simulink model "SatSIM_revAgustus16_01_R2013a"  (R2013a)
settings: Solver=ode15s  StartTime=0.0  StopTime=6000  RelTol=1e-3
values from neighbouring files (symbols this model uses):
  dfy = d    [dfy.m]
  s = sin(ir)    [B_dipole_June16_2.m]    (also in LTC_to_NED.m = sin(e); LTC_to_NED_edit.m = sin(e); TimeConverter.m = fix(sec); read_epoch.m = ((e-h)*60)-min)
undefined symbols (not defined in the file or in its folder): B_dipole_June16_2, DCM_ROI, deg, Earth_MagField_may16_Rev4, InertiaMoment3, LTC_to_NED_edit, rad, read_epochS, sec_to_ymdhms2, SimpleB5
libraries: aerolibconvert2 x13, aerolibutil x7, aerolibtransform2 x4, dspmtrx3 x3, vrlib x2, aerolibanim x1
(part 1 of 2)
settings Model: Creator=Ali Muksin  LastModifiedBy=Ali Muksin
settings DebuggingCC: UnderspecifiedInitializationDetection=Simplified  MergeDetectMultiDrivingBlocksExec=error  SolverPrmCheckMsg=none  FrameProcessingCompatibilityMsg=error  StateNameClashWarn=none
settings GRTTargetCC: CodeReplacementLibrary=C89/C90 (ANSI)

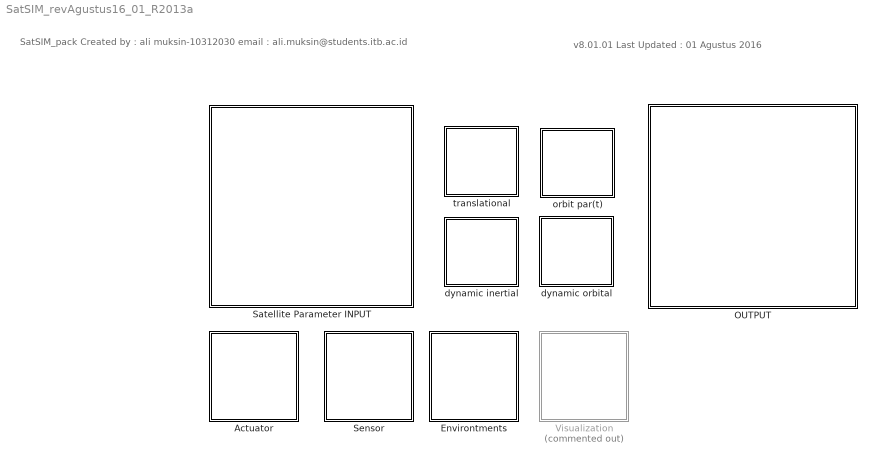
== system SatSIM_revAgustus16_01_R2013a ==
  note: SatSIM_pack
      | Created by : ali muksin-10312030
      | email : ali.muksin@students.itb.ac.id
  note: v8.01.01
      | Last Updated : 01 Agustus 2016
  Actuator : Subsystem
  Environtments : Subsystem
  OUTPUT : Subsystem
  Satellite Parameter INPUT : Subsystem
  Sensor : Subsystem
  Visualization : Subsystem  Commented=on
  dynamic inertial : Subsystem
  dynamic orbital : Subsystem
  orbit par(t) : Subsystem
  translational : Subsystem

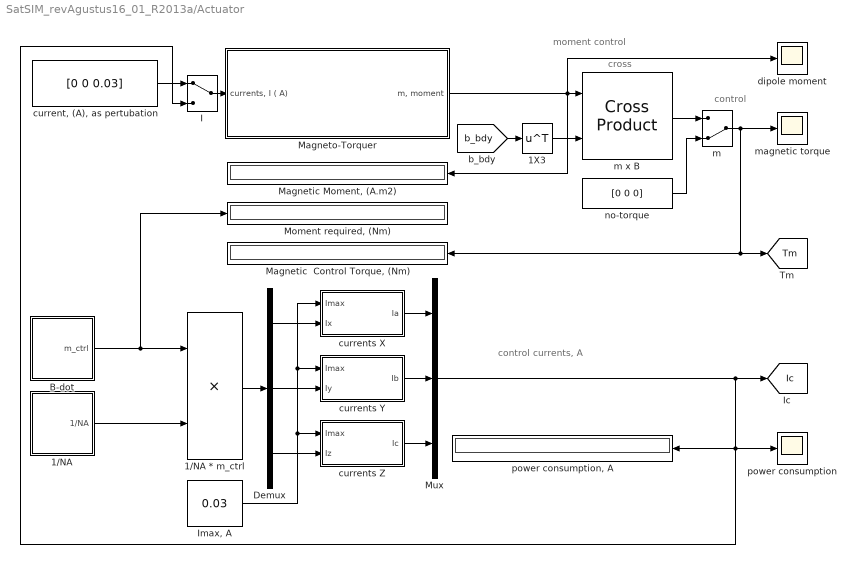
== system SatSIM_revAgustus16_01_R2013a/Actuator ==
  note: control currents, A
  note: moment control
  note: cross
  note: control
  1/NA : Subsystem
  1/NA * m_ctrl : Product
  1X3 : Math  Operator=transpose  SaturateOnIntegerOverflow=on
  B-dot : Subsystem
  Demux : Demux  Outputs=3
  I : ManualSwitch
  "Imax, A" : Constant  Value=0.03
  "Magnetic  Control Torque, (Nm)" : Display
  "Magnetic Moment, (A.m2) " : Display
  Magneto-Torquer : Subsystem
  "Moment required, (Nm)" : Display
  Mux : Mux  Inputs=3
  "current, (A), as pertubation" : Constant  Value=[0 0 0.03]
  currents X : MATLAB Function  TreatAsAtomicUnit=on
      settings: PermitHierarchicalResolution=ParametersOnly
  currents Y : MATLAB Function  TreatAsAtomicUnit=on
      settings: PermitHierarchicalResolution=ParametersOnly
  currents Z : MATLAB Function  TreatAsAtomicUnit=on
      settings: PermitHierarchicalResolution=ParametersOnly
  dipole moment : Scope
      settings: YMin=-0.11  YMax=0.11  SaveName=ScopeData5
  m : ManualSwitch  CurrentSetting=0
  m x B : vrlib/Utilities/Cross Product
  magnetic torque : Scope
      settings: YMin=-2.5e-08  YMax=2.75e-08  SaveName=ScopeData6
  no-torque : Constant  Value=[0 0 0]
  power consumption : Scope
      settings: YMin=-7e-06  YMax=6e-06  SaveName=ScopeData8
  "power consumption, A" : Display
  tag scope: Ic=global, Tm=global
  wires:
  no-torque/1 -> m/2
  m x B/1 -> m/1
  I/1 -> Magneto-Torquer/1("currents, I ( A)")
  "current, (A), as pertubation"/1 -> I/1
  [b_bdy] -> 1X3/1
  1X3/1 -> m x B/2
  1/NA/1(1/NA) -> 1/NA * m_ctrl/2
  currents X/1(Ia) -> Mux/1
  currents Y/1(Ib) -> Mux/2
  currents Z/1(Ic) -> Mux/3
  1/NA * m_ctrl/1 -> Demux/1
  Magneto-Torquer/1("m, moment") -> dipole moment/1, "Magnetic Moment, (A.m2) "/1, m x B/1
  B-dot/1(m_ctrl) -> 1/NA * m_ctrl/1, "Moment required, (Nm)"/1
  "Imax, A"/1 -> currents Z/1(Imax), currents Y/1(Imax), currents X/1(Imax)
  Demux/1 -> currents X/2(Ix)
  Demux/2 -> currents Y/2(Iy)
  Demux/3 -> currents Z/2(Iz)
  Mux/1 -> I/2, power consumption/1, "power consumption, A"/1, [Ic]
  m/1 -> "Magnetic  Control Torque, (Nm)"/1, [Tm], magnetic torque/1

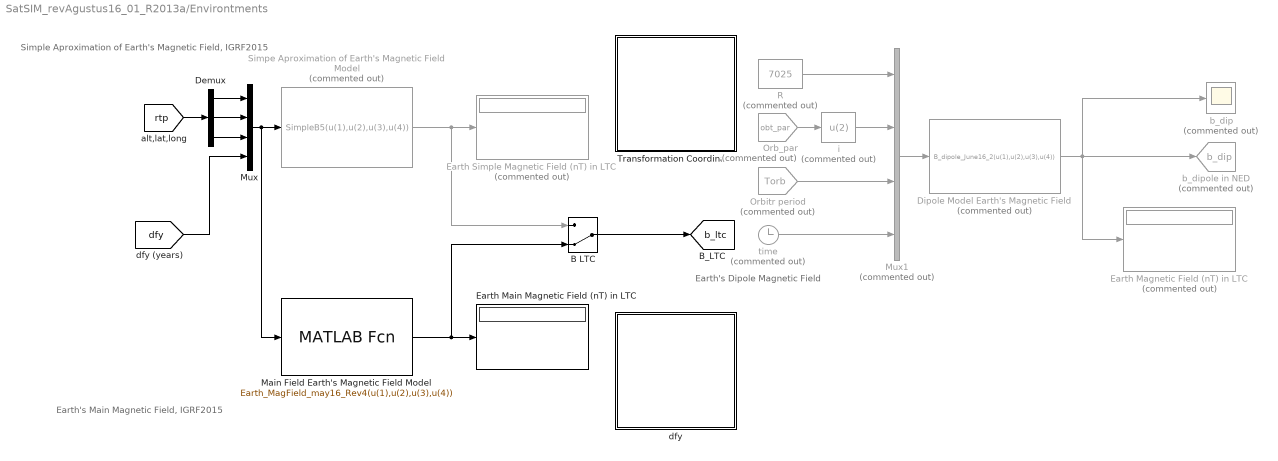
== system SatSIM_revAgustus16_01_R2013a/Environtments ==
  note: Simple Aproximation of Earth's Magnetic Field, IGRF2015
  note: Earth's Main Magnetic Field, IGRF2015
  note: Earth's Dipole Magnetic Field
  B LTC : ManualSwitch  CurrentSetting=0
  Demux : Demux  Outputs=3
  Dipole Model Earth's Magnetic Field : MATLABFcn  Commented=on  MATLABFcn=B_dipole_June16_2(u(1),u(2),u(3),u(4))  Output1D=off
  Earth Magnetic Field (nT) in LTC : Display  Commented=on
  Earth Main Magnetic Field (nT) in LTC : Display
  Earth Simple Magnetic Field (nT) in LTC : Display  Commented=on
  Main Field Earth's Magnetic Field Model : MATLABFcn  MATLABFcn=Earth_MagField_may16_Rev4(u(1),u(2),u(3),u(4))  Output1D=off
  Mux : Mux
  Mux1 : Mux  Commented=on
  Orb_par : From  Commented=on  GotoTag=obt_par  TagVisibility=global
  Orbitr period : From  Commented=on  GotoTag=Torb  TagVisibility=global
  R : Constant  Commented=on  Value=7025
  Simpe Aproximation of Earth's Magnetic Field Model : MATLABFcn  Commented=on  MATLABFcn=SimpleB5(u(1),u(2),u(3),u(4))  Output1D=off
  Transformation Coordinate : Subsystem
  b_dip : Scope  Commented=on
      settings: YMin=2.5e+12  YMax=3.25e+13  SaveName=ScopeData9
  b_dipole in NED : Goto  Commented=on  GotoTag=b_dip  TagVisibility=global
  dfy : Subsystem
  i : Fcn  Commented=on  Expr=u(2)
  time : Clock  Commented=on
  tag scope: b_ltc=global
  wires:
  Simpe Aproximation of Earth's Magnetic Field Model/1 -> B LTC/1, Earth Simple Magnetic Field (nT) in LTC/1
  Demux/1 -> Mux/1
  Demux/2 -> Mux/2
  Demux/3 -> Mux/3
  [dfy] -> Mux/4
  Mux/1 -> Main Field Earth's Magnetic Field Model/1, Simpe Aproximation of Earth's Magnetic Field Model/1
  Main Field Earth's Magnetic Field Model/1 -> B LTC/2, Earth Main Magnetic Field (nT) in LTC/1
  B LTC/1 -> [b_ltc]
  [rtp] -> Demux/1
  R/1 -> Mux1/1
  i/1 -> Mux1/2
  Orb_par/1 -> i/1
  Mux1/1 -> Dipole Model Earth's Magnetic Field/1
  Dipole Model Earth's Magnetic Field/1 -> Earth Magnetic Field (nT) in LTC/1, b_dip/1, b_dipole in NED/1
  Orbitr period/1 -> Mux1/3
  time/1 -> Mux1/4

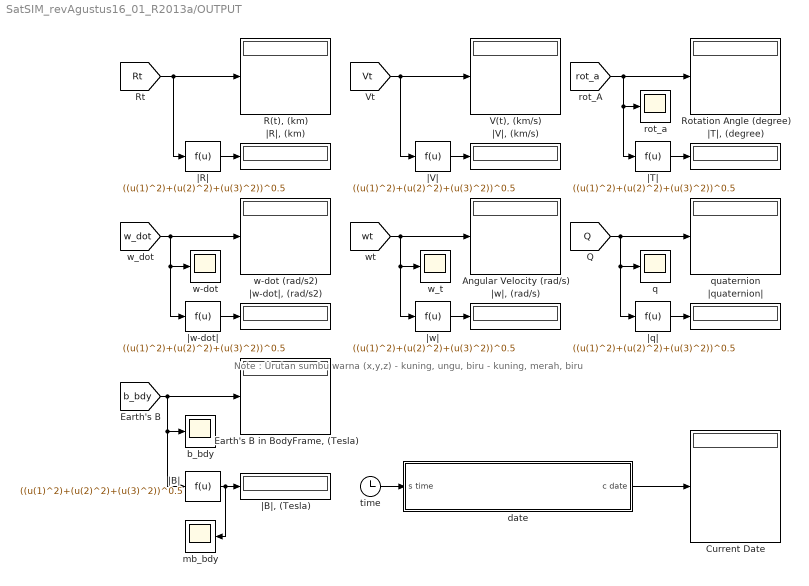
== system SatSIM_revAgustus16_01_R2013a/OUTPUT ==
  note: Note : Urutan sumbu warna (x,y,z)
      | 		- kuning, ungu, biru
      | 		- kuning, merah, biru
  Angular Velocity (rad/s) : Display
  Current Date : Display
  "Earth's B in BodyFrame, (Tesla)" : Display
  "R(t), (km)" : Display
  Rotation Angle (degree) : Display
  "V(t), (km/s)" : Display
  b_bdy : Scope
      settings: YMin=-3.5e-05  YMax=5e-05  SaveName=ScopeData3
  date : Subsystem
  mb_bdy : Scope
      settings: YMin=4.177e-05  YMax=4.1855e-05  SaveName=ScopeData4
  q : Scope
      settings: YMin=-0.8  YMax=0.8  SaveName=ScopeData12
  quaternion : Display
  rot_a : Scope
      settings: YMin=-200  YMax=200
  time : Clock
  w-dot : Scope
      settings: YMin=-0.0006  YMax=5e-05  SaveName=ScopeData13
  w-dot (rad/s2) : Display
  w_t : Scope
      settings: YMin=-0.015  YMax=0.035
  |B| : Fcn  Expr=((u(1)^2)+(u(2)^2)+(u(3)^2))^0.5
  "|B|, (Tesla)" : Display
  |R| : Fcn  Expr=((u(1)^2)+(u(2)^2)+(u(3)^2))^0.5
  "|R|, (km) " : Display
  |T| : Fcn  Expr=((u(1)^2)+(u(2)^2)+(u(3)^2))^0.5
  "|T|, (degree)" : Display
  |V| : Fcn  Expr=((u(1)^2)+(u(2)^2)+(u(3)^2))^0.5
  "|V|, (km/s)" : Display
  |quaternion| : Display
  |q| : Fcn  Expr=((u(1)^2)+(u(2)^2)+(u(3)^2))^0.5
  |w-dot| : Fcn  Expr=((u(1)^2)+(u(2)^2)+(u(3)^2))^0.5
  "|w-dot|, (rad/s2)" : Display
  |w| : Fcn  Expr=((u(1)^2)+(u(2)^2)+(u(3)^2))^0.5
  "|w|, (rad/s)" : Display
  wires:
  [rot_a] -> |T|/1, rot_a/1, Rotation Angle (degree)/1
  [Rt] -> |R|/1, "R(t), (km)"/1
  [Vt] -> |V|/1, "V(t), (km/s)"/1
  |V|/1 -> "|V|, (km/s)"/1
  [wt] -> |w|/1, w_t/1, Angular Velocity (rad/s)/1
  |R|/1 -> "|R|, (km) "/1
  |T|/1 -> "|T|, (degree)"/1
  |w|/1 -> "|w|, (rad/s)"/1
  date/1(c date) -> Current Date/1
  time/1 -> date/1(s time)
  |B|/1 -> mb_bdy/1, "|B|, (Tesla)"/1
  [b_bdy] -> "Earth's B in BodyFrame, (Tesla)"/1, b_bdy/1, |B|/1
  [w_dot] -> w-dot/1, |w-dot|/1, w-dot (rad/s2)/1
  |w-dot|/1 -> "|w-dot|, (rad/s2)"/1
  [Q] -> q/1, |q|/1, quaternion/1
  |q|/1 -> |quaternion|/1

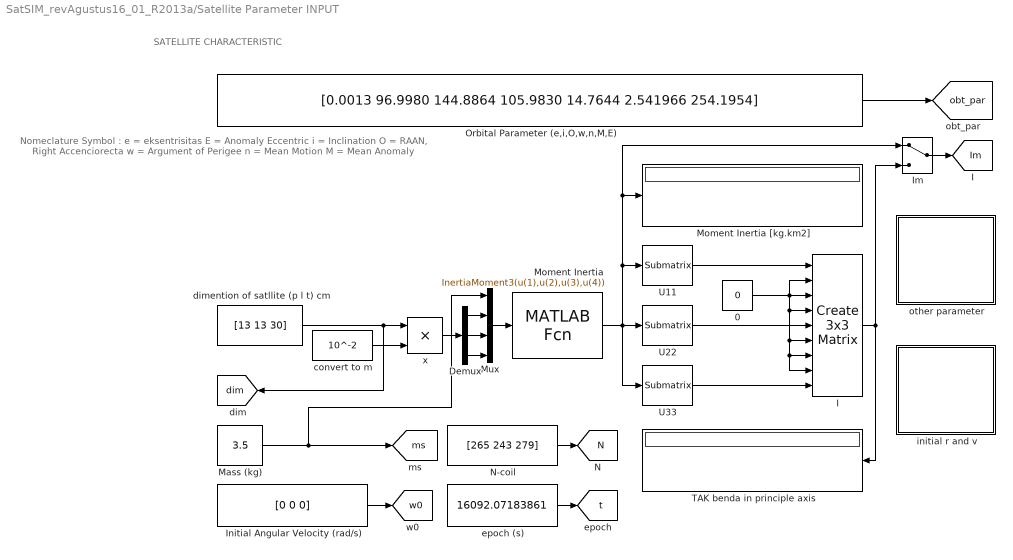
== system SatSIM_revAgustus16_01_R2013a/Satellite Parameter INPUT ==
  note: Nomeclature Symbol :
      | e	= eksentrisitas						  E	= Anomaly Eccentric
      | i	= Inclination
      | O	= RAAN, Right Accenciorecta
      | w	= Argument of Perigee
      | n	= Mean Motion
      | M	= Mean Anomaly
  note: SATELLITE CHARACTERISTIC
  0 : Constant  Value=0
  Demux : Demux  Outputs=3
  "I " : aerolibutil/Create 3x3 Matrix
  Im : ManualSwitch
  Initial Angular Velocity (rad/s) : Constant  Value=[0 0 0]
  Mass (kg) : Constant  Value=3.5
  Moment Inertia : MATLABFcn  MATLABFcn=InertiaMoment3(u(1),u(2),u(3),u(4))  Output1D=off
  Moment Inertia [kg.km2] : Display
  Mux : Mux
  N-coil : Constant  Value=[265 243 279]
  Orbital Parameter (e,i,O,w,n,M,E) : Constant  Value=[0.0013 96.9980 144.8864 105.9830 14.7644 2.541966 254.1954]  VectorParams1D=off
  TAK benda in principle axis : Display
  U11 : dspmtrx3/Submatrix  RowSpan=One row  RowStartMode=First  RowStartIndex=1  RowEndMode=Last  RowEndIndex=1  ColSpan=One column  ColStartMode=First  ColStartIndex=1  ColEndMode=Last  ColEndIndex=1
  U22 : dspmtrx3/Submatrix  RowSpan=One row  RowStartMode=Middle  RowStartIndex=1  RowEndMode=Last  RowEndIndex=1  ColSpan=One column  ColStartMode=Middle  ColStartIndex=1  ColEndMode=Last  ColEndIndex=1
  U33 : dspmtrx3/Submatrix  RowSpan=One row  RowStartMode=Last  RowStartIndex=1  RowEndMode=Last  RowEndIndex=1  ColSpan=One column  ColStartMode=Last  ColStartIndex=1  ColEndMode=Last  ColEndIndex=1
  convert to m : Constant  Value=10^-2
  dimention of satllite (p l t) cm : Constant  Value=[13 13 30]
  epoch (s) : Constant  Value=16092.07183861
  initial r and v : Subsystem
  other parameter : Subsystem
  x : Product
  tag scope: Im=global, N=global, dim=global, ms=global, obt_par=global, t=global, w0=global
  wires:
  dimention of satllite (p l t) cm/1 -> [dim], x/1
  Mass (kg)/1 -> Mux/1, [ms]
  Orbital Parameter (e,i,O,w,n,M,E)/1 -> [obt_par]
  N-coil/1 -> [N]
  Initial Angular Velocity (rad/s)/1 -> [w0]
  epoch (s)/1 -> [t]
  Moment Inertia/1 -> U33/1, U22/1, U11/1, Im/1, Moment Inertia [kg.km2]/1
  convert to m/1 -> x/2
  x/1 -> Demux/1
  0/1 -> "I "/3, "I "/7, "I "/8, "I "/6, "I "/4, "I "/2
  "I "/1 -> Im/2, TAK benda in principle axis/1
  U11/1 -> "I "/1
  U22/1 -> "I "/5
  U33/1 -> "I "/9
  Demux/1 -> Mux/2
  Demux/2 -> Mux/3
  Demux/3 -> Mux/4
  Mux/1 -> Moment Inertia/1
  Im/1 -> [Im]

== system SatSIM_revAgustus16_01_R2013a/Sensor ==
  note: 1 nT = 1*10^-9 T
  Earth Magnetic Field (T) in ECI : Display
  RIB^-1 : aerolibutil/Invert  3x3 Matrix
  Transform Inertia to Body : Product  Multiplication=Matrix(*)
  nT to T : Constant  Value=1/10^9
  x : Product
  tag scope: b_bdy=global
  wires:
  nT to T/1 -> x/2
  x/1 -> Earth Magnetic Field (T) in ECI/1, Transform Inertia to Body/2
  Transform Inertia to Body/1 -> [b_bdy]
  [RIB] -> RIB^-1/1
  RIB^-1/1 -> Transform Inertia to Body/1
  [b_eci] -> x/1

== system SatSIM_revAgustus16_01_R2013a/Visualization ==
  note: Output - Animation
  6DoF Animation : aerolibanim/6DoF Animation  u1=[-15000 15000 -15000 15000 -15000 15000]  u2=0.1  u3=2000  u4=[0 0 0]  u5=Fixed position  u6=[60000 120000 60000]  u7=10  u8=off
  wires:
  [Rt] -> 6DoF Animation/1  "r_vector"
  [rot_a] -> 6DoF Animation/2

== system SatSIM_revAgustus16_01_R2013a/dynamic inertial ==
  note: Body To Inertial Frame
      | or ECI
  note: Euler Axis
      | 3x1
  note: Teta (degree)
  Angle Conversion : aerolibconvert2/Angle Conversion  IU=rad  OU=deg
  Attitude Dynamic : Subsystem
  DCM RIB : Display
  DCM to Euler Parameter : MATLAB Function  TreatAsAtomicUnit=on
      settings: PermitHierarchicalResolution=ParametersOnly
  Demux3 : Demux  Outputs=3
  Euler Parameter : Display
  Mux1 : Mux  Inputs=3
  Quaternions to Rotation Angles : aerolibtransform2/Quaternions to Rotation Angles  rotationOrder=ZYX
  Rotation Angle (degree) : Display
  Rotation Angles to Direction Cosine Matrix : aerolibtransform2/Rotation Angles to Direction Cosine Matrix  rotationOrder=ZYX
  w(t) to Quaternion : Subsystem
  tag scope: E_par=global, RIB=global, rot_a=global
  wires:
  Mux1/1 -> Rotation Angles to Direction Cosine Matrix/1
  Demux3/2 -> Mux1/2
  Demux3/1 -> Mux1/1
  Angle Conversion/1 -> Rotation Angle (degree)/1, Demux3/1, [rot_a]
  Rotation Angles to Direction Cosine Matrix/1 -> DCM to Euler Parameter/1(DCM), DCM RIB/1, [RIB]
  Demux3/3 -> Mux1/3
  Quaternions to Rotation Angles/1 -> Angle Conversion/1
  Attitude Dynamic/1(wt) -> w(t) to Quaternion/1(wt)
  w(t) to Quaternion/1(q) -> Quaternions to Rotation Angles/1
  DCM to Euler Parameter/1(B) -> Euler Parameter/1, [E_par]

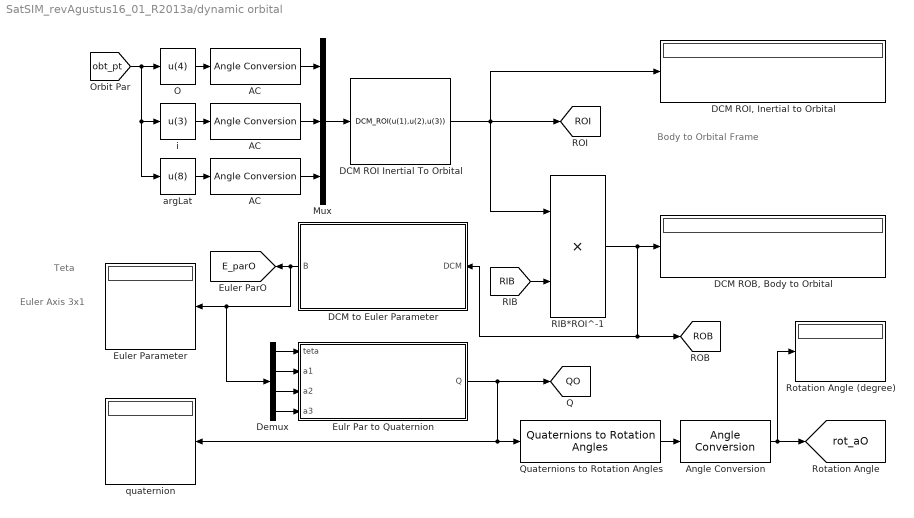
== system SatSIM_revAgustus16_01_R2013a/dynamic orbital ==
  note: Euler Axis
      | 3x1
  note: Teta
  note: Body to
      | Orbital Frame
  AC : aerolibconvert2/Angle Conversion  IU=rad  OU=deg
  "AC " : aerolibconvert2/Angle Conversion  IU=rad  OU=deg
  "AC " : aerolibconvert2/Angle Conversion  IU=rad  OU=deg
  Angle Conversion : aerolibconvert2/Angle Conversion  IU=rad  OU=deg
  "DCM ROB, Body to Orbital" : Display
  DCM ROI Inertial To Orbital : MATLABFcn  MATLABFcn=DCM_ROI(u(1),u(2),u(3))  Output1D=off
  "DCM ROI, Inertial to Orbital" : Display
  DCM to Euler Parameter : MATLAB Function  TreatAsAtomicUnit=on
      settings: PermitHierarchicalResolution=ParametersOnly
  Demux : Demux
  Euler Parameter : Display
  Eulr Par to Quaternion : MATLAB Function  TreatAsAtomicUnit=on
      settings: PermitHierarchicalResolution=ParametersOnly
  Mux : Mux  Inputs=3
  O : Fcn  Expr=u(4)
  Quaternions to Rotation Angles : aerolibtransform2/Quaternions to Rotation Angles  rotationOrder=ZYX
  RIB*ROI^-1 : Product
  Rotation Angle (degree) : Display
  argLat : Fcn  Expr=u(8)
  i : Fcn  Expr=u(3)
  quaternion : Display
  tag scope: E_parO=global, QO=global, ROB=global, ROI=global, rot_aO=global
  wires:
  AC/1 -> Mux/1
  Mux/1 -> DCM ROI Inertial To Orbital/1
  O/1 -> AC/1
  "AC "/1 -> Mux/3
  argLat/1 -> "AC "/1
  i/1 -> "AC "/1
  "AC "/1 -> Mux/2
  [obt_pt] -> argLat/1, i/1, O/1
  DCM ROI Inertial To Orbital/1 -> RIB*ROI^-1/1, "DCM ROI, Inertial to Orbital"/1, [ROI]
  RIB*ROI^-1/1 -> [ROB], DCM to Euler Parameter/1(DCM), "DCM ROB, Body to Orbital"/1
  DCM to Euler Parameter/1(B) -> Euler Parameter/1, Demux/1, [E_parO]
  Demux/1 -> Eulr Par to Quaternion/1(teta)
  Demux/2 -> Eulr Par to Quaternion/2(a1)
  Demux/3 -> Eulr Par to Quaternion/3(a2)
  Demux/4 -> Eulr Par to Quaternion/4(a3)
  Quaternions to Rotation Angles/1 -> Angle Conversion/1
  Eulr Par to Quaternion/1(Q) -> Quaternions to Rotation Angles/1, quaternion/1, [QO]
  Angle Conversion/1 -> Rotation Angle (degree)/1, [rot_aO]
  [RIB] -> RIB*ROI^-1/2

== system SatSIM_revAgustus16_01_R2013a/orbit par(t) ==
  note: Output	:
      | %------------------------------------------------------------------%
      | p			= Semilatus Rectum (km)
      | e			= Eccentricity Magnitude
      | i			= Inclination (rad)
      | O			= Right Ascention of the ascending node (rad)
      | o			= Argument of perigee (rad)
      | nu			= True Anomaly (rad)
      | truLon	= True Longitude (rad)
      | argLat	= Argument of Latitude (rad)
      | lonPer	= Longitude of Periapse (rad)
      | mu		= Gravitational Constant
  Mux : Mux  Inputs=10
  Orbital Parameter (t) : Display
  R(t) and V(t) to Orbital Parameter : MATLAB Function  TreatAsAtomicUnit=on
      settings: PermitHierarchicalResolution=ParametersOnly
  tag scope: obt_pt=global
  wires:
  R(t) and V(t) to Orbital Parameter/3(i) -> Mux/3
  [Vt] -> R(t) and V(t) to Orbital Parameter/2(v)
  R(t) and V(t) to Orbital Parameter/5(o) -> Mux/5
  [u] -> R(t) and V(t) to Orbital Parameter/3(mu)
  R(t) and V(t) to Orbital Parameter/1(a) -> Mux/1
  R(t) and V(t) to Orbital Parameter/4(O) -> Mux/4
  R(t) and V(t) to Orbital Parameter/6(nu) -> Mux/6
  R(t) and V(t) to Orbital Parameter/7(truLon) -> Mux/7
  R(t) and V(t) to Orbital Parameter/8(argLat) -> Mux/8
  R(t) and V(t) to Orbital Parameter/9(lonPer) -> Mux/9
  R(t) and V(t) to Orbital Parameter/10(p) -> Mux/10
  Mux/1 -> [obt_pt], Orbital Parameter (t)/1
  R(t) and V(t) to Orbital Parameter/2(eMag) -> Mux/2
  [Rt] -> R(t) and V(t) to Orbital Parameter/1(r)

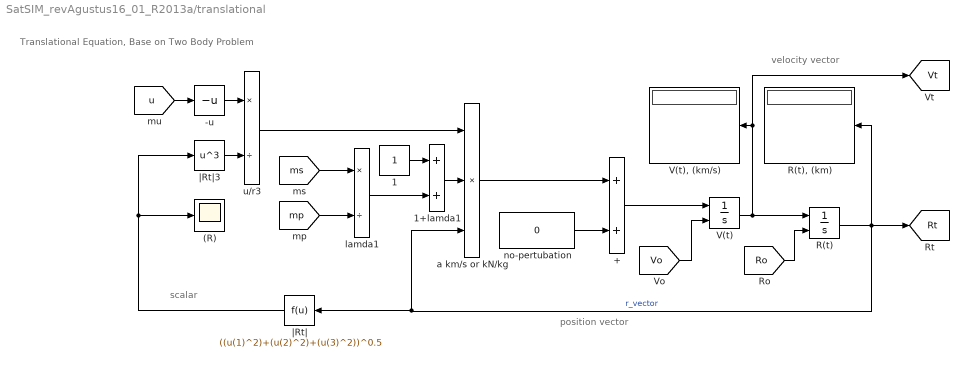
== system SatSIM_revAgustus16_01_R2013a/translational ==
  note: position vector
  note: velocity vector
  note: scalar
  note: Translational Equation, Base on Two Body Problem
  (R) : Scope
      settings: YMin=7165  YMax=7230  SaveName=ScopeData2
  + : Sum
  -u : UnaryMinus
  1 : Constant
  1+lamda1 : Sum
  R(t) : Integrator  InitialConditionSource=external
  "R(t), (km)" : Display
  V(t) : Integrator  InitialConditionSource=external
  "V(t), (km/s)" : Display
  a km/s or kN/kg : Product  Inputs=3
  lamda1 : Product  Inputs=*/
  no-pertubation : Constant  Value=0
  u/r3 : Product  Inputs=*/
  |Rt| : Fcn  Expr=((u(1)^2)+(u(2)^2)+(u(3)^2))^0.5
  |Rt|3 : Fcn  Expr=u^3
  tag scope: Rt=global, Vt=global
  wires:
  [Ro] -> R(t)/2
  V(t)/1 -> "V(t), (km/s)"/1, [Vt], R(t)/1
  R(t)/1 -> |Rt|/1, a km/s or kN/kg/3, "R(t), (km)"/1, [Rt]  "r_vector"
  +/1 -> V(t)/1
  [Vo] -> V(t)/2
  [u] -> -u/1
  no-pertubation/1 -> +/2
  |Rt|3/1 -> u/r3/2
  a km/s or kN/kg/1 -> +/1
  -u/1 -> u/r3/1
  u/r3/1 -> a km/s or kN/kg/1
  [ms] -> lamda1/1
  [mp] -> lamda1/2
  lamda1/1 -> 1+lamda1/2
  1/1 -> 1+lamda1/1
  1+lamda1/1 -> a km/s or kN/kg/2
  |Rt|/1 -> (R)/1, |Rt|3/1

== system SatSIM_revAgustus16_01_R2013a/Actuator/1//NA ==
  note: NA
  note: t
  note: l
  note: p
  1 : Constant
  "1/NA " : Product  Inputs=*/
  Ax : Product
  Ay : Product
  Az : Product
  Demux : Demux  Outputs=3
  Demux1 : Demux  Outputs=3
  Mux : Mux  Inputs=3
  convert to m : Constant  Value=10^(-2)
  lt : Product
  pl : Product
  pt : Product
  x : Product
  1/NA : Outport
  wires:
  Demux1/1 -> pt/1, pl/1
  Demux/2 -> Ay/1
  Demux/1 -> Ax/1
  Demux1/2 -> pl/2, lt/1
  Ay/1 -> Mux/2
  Mux/1 -> "1/NA "/2
  pl/1 -> Az/2
  x/1 -> Demux1/1
  [N] -> Demux/1
  convert to m/1 -> x/2
  Ax/1 -> Mux/1
  Az/1 -> Mux/3
  [dim] -> x/1
  Demux/3 -> Az/1
  Demux1/3 -> lt/2, pt/2
  pt/1 -> Ax/2
  lt/1 -> Ay/2
  1/1 -> "1/NA "/1
  "1/NA "/1 -> 1/NA/1

== system SatSIM_revAgustus16_01_R2013a/Actuator/B-dot ==
  note: b-dot
  " " : Integrator
  -kd*B-dot : Product  Multiplication=Matrix(*)
  0 : Constant  Value=0
  1X3 : Math  Operator=transpose  SaturateOnIntegerOverflow=on
  Sum : Sum  Inputs=|+-
  control gain : Display
      settings: Format=short_e
  k : Constant  Value=1*(10^1)
  k-dot : aerolibutil/Create 3x3 Matrix
  k-dot/|B| : Product  Inputs=*/
  w x B : vrlib/Utilities/Cross Product
  |B| : Fcn  Expr=((u(1)^2)+(u(2)^2)+(u(3)^2))^0.5
  m_ctrl : Outport
  wires:
  " "/1 -> Sum/2
  w x B/1 -> -kd*B-dot/2, " "/1
  0/1 -> k-dot/8, k-dot/7, k-dot/6, k-dot/4, k-dot/3, k-dot/2
  -kd*B-dot/1 -> m_ctrl/1
  k-dot/1 -> k-dot/|B|/1, control gain/1
  [b_bdy] -> 1X3/1
  1X3/1 -> |B|/1, Sum/1
  k-dot/|B|/1 -> -kd*B-dot/1
  |B|/1 -> k-dot/|B|/2
  [wt] -> w x B/1
  Sum/1 -> w x B/2
  k/1 -> k-dot/9, k-dot/5, k-dot/1

== system SatSIM_revAgustus16_01_R2013a/Actuator/Magneto-Torquer ==
  note: t
  note: l
  note: p
  "currents, I ( A)" : Inport
  Ax : Product  Inputs=3
  Ay : Product  Inputs=3
  Az : Product  Inputs=3
  Demux : Demux  Outputs=3
  Demux1 : Demux  Outputs=3
  Demux2 : Demux  Outputs=3
  Mux : Mux  Inputs=3
  convert to m : Constant  Value=10^(-2)
  lt : Product
  pl : Product
  pt : Product
  x : Product
  "m, moment" : Outport
  wires:
  Ax/1 -> Mux/1
  lt/1 -> Ay/2
  Demux1/1 -> pt/1, pl/1
  Demux1/2 -> pl/2, lt/1
  pt/1 -> Ax/2
  x/1 -> Demux1/1
  [dim] -> x/1
  pl/1 -> Az/2
  Demux/3 -> Az/1
  Ay/1 -> Mux/2
  Mux/1 -> "m, moment"/1
  Demux/1 -> Ax/1
  Demux1/3 -> lt/2, pt/2
  Demux/2 -> Ay/1
  [N] -> Demux/1
  convert to m/1 -> x/2
  "currents, I ( A)"/1 -> Demux2/1
  Az/1 -> Mux/3
  Demux2/3 -> Az/3
  Demux2/1 -> Ax/3
  Demux2/2 -> Ay/3

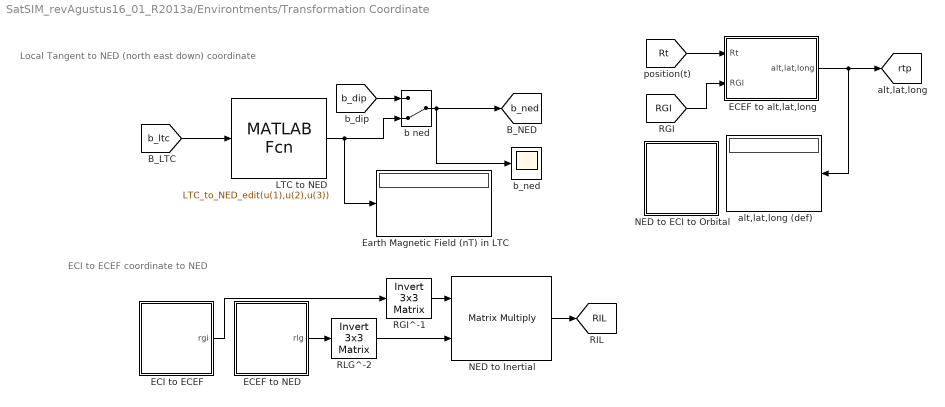
== system SatSIM_revAgustus16_01_R2013a/Environtments/Transformation Coordinate ==
  note: Local Tangent to NED (north east down) coordinate
  note: ECI to ECEF coordinate to NED
  ECEF to NED : Subsystem
  ECEF to alt,lat,long : Subsystem
  ECI to ECEF : Subsystem
  Earth Magnetic Field (nT) in LTC : Display
  LTC to NED : MATLABFcn  MATLABFcn=LTC_to_NED_edit(u(1),u(2),u(3))  Output1D=off
  NED to ECI to Orbital : Subsystem
  NED to Inertial : Product  Multiplication=Matrix(*)
  RGI^-1 : aerolibutil/Invert  3x3 Matrix
  RLG^-2 : aerolibutil/Invert  3x3 Matrix
  alt,lat,long (def) : Display
  b ned : ManualSwitch  CurrentSetting=0
  b_ned : Scope
      settings: ShowLegends=on  YMin=-4e-05  YMax=4e-05  SaveName=ScopeData10
  tag scope: RIL=global, b_ned=global, rtp=global
  wires:
  [b_ltc] -> LTC to NED/1
  LTC to NED/1 -> b ned/2, Earth Magnetic Field (nT) in LTC/1
  NED to Inertial/1 -> [RIL]
  ECEF to alt,lat,long/1(alt,lat,long) -> alt,lat,long (def)/1, [rtp]
  [Rt] -> ECEF to alt,lat,long/1(Rt)
  [RGI] -> ECEF to alt,lat,long/2(RGI)
  RLG^-2/1 -> NED to Inertial/2
  ECEF to NED/1(rlg) -> RLG^-2/1
  RGI^-1/1 -> NED to Inertial/1
  ECI to ECEF/1(rgi) -> RGI^-1/1
  b ned/1 -> b_ned/1, [b_ned]
  [b_dip] -> b ned/1

== system SatSIM_revAgustus16_01_R2013a/Environtments/dfy ==
  note: day fraction as fungtion of years
  note: ymd
  note: dmy
  Demux3 : Demux  Outputs=3
  Mux1 : Mux  Inputs=2
  Mux2 : Mux  Inputs=3
  day fraction : MATLABFcn  MATLABFcn=dfy(u(1),u(2),u(3),u(4),u(5),u(6))  Output1D=off
  dfy (years) : Display
  tag scope: dfy=global
  wires:
  [time] -> Mux1/2
  day fraction/1 -> [dfy], dfy (years)/1
  [date] -> Demux3/1
  Demux3/2 -> Mux2/2
  Mux2/1 -> Mux1/1
  Demux3/1 -> Mux2/3
  Mux1/1 -> day fraction/1
  Demux3/3 -> Mux2/1

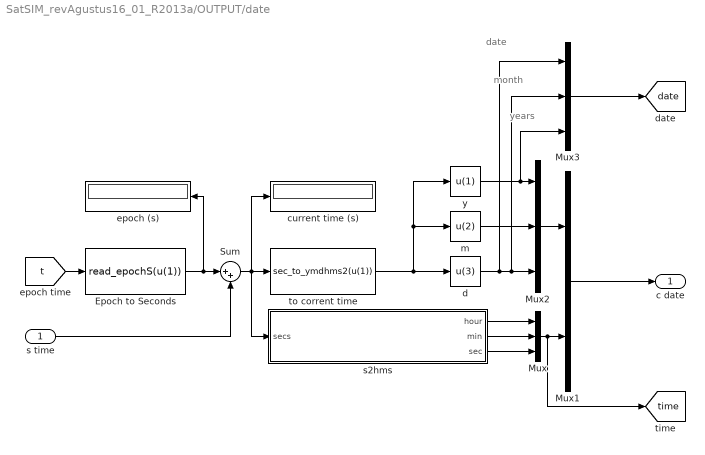
== system SatSIM_revAgustus16_01_R2013a/OUTPUT/date ==
  note: date
  note: month
  note: years
  s time : Inport
  Epoch to Seconds : MATLABFcn  MATLABFcn=read_epochS(u(1))  Output1D=off
  Mux : Mux  Inputs=3
  Mux1 : Mux  Inputs=2
  Mux2 : Mux  Inputs=3
  Mux3 : Mux  Inputs=3
  Sum : Sum  Inputs=|++
  current time (s) : Display
  d : Fcn  Expr=u(3)
  epoch (s) : Display
  m : Fcn  Expr=u(2)
  s2hms : MATLAB Function  TreatAsAtomicUnit=on
      settings: PermitHierarchicalResolution=ParametersOnly
  to corrent time : MATLABFcn  MATLABFcn=sec_to_ymdhms2(u(1))
  y : Fcn  Expr=u(1)
  c date : Outport
  tag scope: date=global, time=global
  wires:
  Sum/1 -> s2hms/1(secs), to corrent time/1, current time (s)/1
  s2hms/3(sec) -> Mux/3
  s2hms/1(hour) -> Mux/1
  s2hms/2(min) -> Mux/2
  [t] -> Epoch to Seconds/1
  Epoch to Seconds/1 -> Sum/1, epoch (s)/1
  Mux1/1 -> c date/1
  to corrent time/1 -> m/1, y/1, d/1
  Mux/1 -> [time], Mux1/2
  Mux2/1 -> Mux1/1
  y/1 -> Mux3/3, Mux2/1
  m/1 -> Mux2/2
  s time/1 -> Sum/2
  d/1 -> Mux3/1, Mux3/2, Mux2/3
  Mux3/1 -> [date]

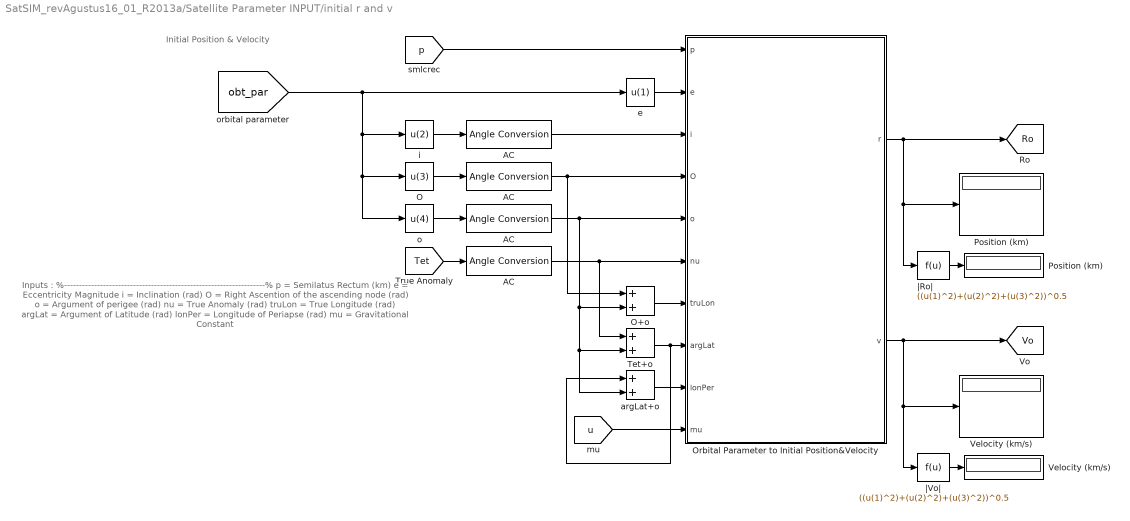
== system SatSIM_revAgustus16_01_R2013a/Satellite Parameter INPUT/initial r and v ==
  note: Initial Position & Velocity
  note: Inputs	:
      | %-------------------------------------------------------------------%
      | p			= Semilatus Rectum (km)
      | e			= Eccentricity Magnitude
      | i			= Inclination (rad)
      | O			= Right Ascention of the ascending node (rad)
      | o			= Argument of perigee (rad)
      | nu			= True Anomaly (rad)
      | truLon	= True Longitude (rad)
      | argLat	= Argument of Latitude (rad)
      | lonPer	= Longitude of Periapse (rad)
      | mu		= Gravitational Constant
  AC : aerolibconvert2/Angle Conversion  IU=deg  OU=rad
  "AC " : aerolibconvert2/Angle Conversion  IU=deg  OU=rad
  "AC " : aerolibconvert2/Angle Conversion  IU=deg  OU=rad
  "AC " : aerolibconvert2/Angle Conversion  IU=deg  OU=rad
  O : Fcn  Expr=u(3)
  O+o : Sum
  Orbital Parameter to Initial Position&Velocity : MATLAB Function  TreatAsAtomicUnit=on
      settings: PermitHierarchicalResolution=ParametersOnly
  Position (km) : Display
  "Position (km) " : Display
  Tet+o : Sum
  Velocity (km/s) : Display
  "Velocity (km/s) " : Display
  argLat+o : Sum
  e : Fcn  Expr=u(1)
  i : Fcn  Expr=u(2)
  o : Fcn  Expr=u(4)
  |Ro| : Fcn  Expr=((u(1)^2)+(u(2)^2)+(u(3)^2))^0.5
  |Vo| : Fcn  Expr=((u(1)^2)+(u(2)^2)+(u(3)^2))^0.5
  tag scope: Ro=global, Vo=global
  wires:
  Orbital Parameter to Initial Position&Velocity/1(r) -> |Ro|/1, Position (km)/1, [Ro]
  [p] -> Orbital Parameter to Initial Position&Velocity/1(p)
  e/1 -> Orbital Parameter to Initial Position&Velocity/2(e)
  [obt_par] -> e/1, i/1, O/1, o/1
  [u] -> Orbital Parameter to Initial Position&Velocity/10(mu)
  |Ro|/1 -> "Position (km) "/1
  Orbital Parameter to Initial Position&Velocity/2(v) -> |Vo|/1, Velocity (km/s)/1, [Vo]
  |Vo|/1 -> "Velocity (km/s) "/1
  i/1 -> AC/1
  AC/1 -> Orbital Parameter to Initial Position&Velocity/3(i)
  O/1 -> "AC "/1
  "AC "/1 -> Orbital Parameter to Initial Position&Velocity/4(O), O+o/1
  o/1 -> "AC "/1
  "AC "/1 -> O+o/2, Tet+o/2, argLat+o/2, Orbital Parameter to Initial Position&Velocity/5(o)
  "AC "/1 -> Tet+o/1, Orbital Parameter to Initial Position&Velocity/6(nu)
  [Tet] -> "AC "/1
  O+o/1 -> Orbital Parameter to Initial Position&Velocity/7(truLon)
  Tet+o/1 -> argLat+o/1, Orbital Parameter to Initial Position&Velocity/8(argLat)
  argLat+o/1 -> Orbital Parameter to Initial Position&Velocity/9(lonPer)

== system SatSIM_revAgustus16_01_R2013a/Satellite Parameter INPUT/other parameter ==
  Earth's Angular Velocity (rad/s) : Constant  Value=7.2921159 *10^-5
  Earth's Mass (kg) : Constant  Value=5.98*10^24
  Earth's Radius (km) : Constant  Value=6378.148
  G ([KN.km2/kg2) : Constant  Value=6.67*10^-20
  Mux : Mux  Inputs=2
  Semi Major Axis and Semilatus Rectum : Subsystem
  VC : aerolibconvert2/Angular Velocity Conversion  IU=rad/s  OU=deg/s
  mu : Product
  periode : Fcn  Expr=2*pi*(((u(1)^3)/u(2))^0.5)
  "periode, (s)" : Display
  tag scope: G=global, Re=global, Torb=global, mp=global, u=global, wE=global
  wires:
  Earth's Angular Velocity (rad/s)/1 -> VC/1
  mu/1 -> [u]
  VC/1 -> [wE]
  Earth's Radius (km)/1 -> [Re]
  G ([KN.km2/kg2)/1 -> [G], mu/1
  Earth's Mass (kg)/1 -> mu/2, [mp]
  Mux/1 -> periode/1
  [a] -> Mux/1
  [u] -> Mux/2
  periode/1 -> [Torb], "periode, (s)"/1

== system SatSIM_revAgustus16_01_R2013a/dynamic inertial/Attitude Dynamic ==
  note: wt
  note: (rad/s2)
  note: Rotational Equation
  (wx(Iw)+t)*I^-1 : Product  Multiplication=Matrix(*)
  + : Sum  Inputs=+++
  I.Wt : Product  Multiplication=Matrix(*)
  Wt x (I.Wt) : aerolibutil/3x3 Cross Product
  disturbance : Constant  Value=[0.0 0.0 0.0]
  inverse(I) : aerolibutil/Invert  3x3 Matrix
  torque (Nm) : Display
  w-dot : Integrator  InitialConditionSource=external
  w-dot (rad/s2) : Display
  w^t : Math  Operator=transpose  SaturateOnIntegerOverflow=on
  "w^t " : Math  Operator=transpose  SaturateOnIntegerOverflow=on
  wt (rad/s) : Display
  wt : Outport
  tag scope: w_dot=global, wt=global
  wires:
  Wt x (I.Wt)/1 -> +/1
  [w0] -> w-dot/2
  inverse(I)/1 -> (wx(Iw)+t)*I^-1/2
  (wx(Iw)+t)*I^-1/1 -> w-dot (rad/s2)/1, [w_dot], w-dot/1
  [Im] -> I.Wt/1, inverse(I)/1
  +/1 -> torque (Nm)/1, (wx(Iw)+t)*I^-1/1
  w-dot/1 -> "w^t "/1, w^t/1, wt (rad/s)/1, [wt]
  w^t/1 -> Wt x (I.Wt)/1, I.Wt/2
  "w^t "/1 -> wt/1
  disturbance/1 -> +/3
  I.Wt/1 -> Wt x (I.Wt)/2
  [Tm] -> +/2

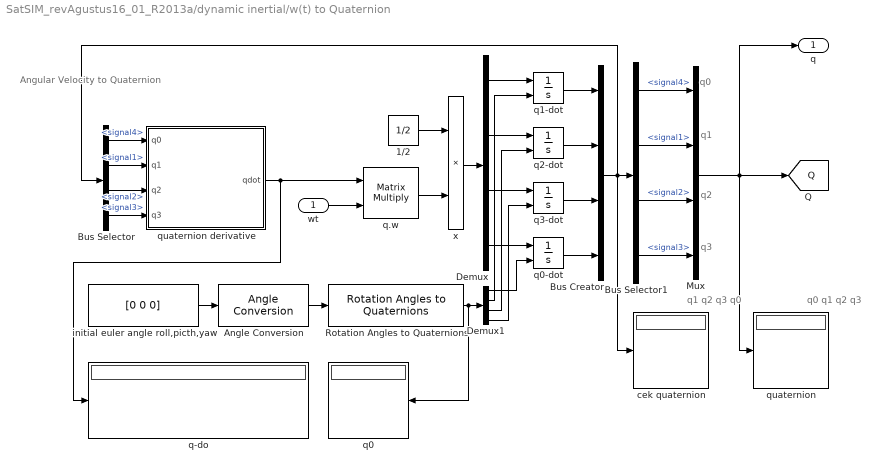
== system SatSIM_revAgustus16_01_R2013a/dynamic inertial/w(t) to Quaternion ==
  note: q1
  note: q0
  note: q0
      | q1
      | q2
      | q3
  note: Angular Velocity to Quaternion
  note: q2
  note: q3
  note: q1
      | q2
      | q3
      | q0
  wt : Inport
  1/2 : Constant  Value=1/2
  Angle Conversion : aerolibconvert2/Angle Conversion  IU=deg  OU=rad
  Bus Creator : BusCreator
  Bus Selector : BusSelector  OutputSignals=signal4,signal1,signal2,signal3
  Bus Selector1 : BusSelector  OutputSignals=signal4,signal1,signal2,signal3
  Demux : Demux
  Demux1 : Demux
  Mux : Mux
  Rotation Angles to Quaternions : aerolibtransform2/Rotation Angles to Quaternions  rotationOrder=ZYX
  cek quaternion : Display
  initial euler angle roll,picth,yaw : Constant  Value=[0 0 0]
  q-do : Display
  q.w : Product  Multiplication=Matrix(*)
  q0 : Display
  q0-dot : Integrator  InitialConditionSource=external
  q1-dot : Integrator  InitialConditionSource=external
  q2-dot : Integrator  InitialConditionSource=external
  q3-dot : Integrator  InitialConditionSource=external
  quaternion : Display
  quaternion derivative : MATLAB Function  TreatAsAtomicUnit=on
      settings: PermitHierarchicalResolution=ParametersOnly
  x : Product
  q : Outport
  tag scope: Q=global
  wires:
  Mux/1 -> q/1, quaternion/1, [Q]
  x/1 -> Demux/1
  Rotation Angles to Quaternions/1 -> q0/1, Demux1/1
  q.w/1 -> x/2
  1/2/1 -> x/1
  quaternion derivative/1(qdot) -> q-do/1, q.w/1
  initial euler angle roll,picth,yaw/1 -> Angle Conversion/1
  Angle Conversion/1 -> Rotation Angles to Quaternions/1
  wt/1 -> q.w/2
  Demux/1 -> q1-dot/1
  Demux/2 -> q2-dot/1
  Demux/3 -> q3-dot/1
  Demux/4 -> q0-dot/1
  q1-dot/1 -> Bus Creator/1
  q2-dot/1 -> Bus Creator/2
  q3-dot/1 -> Bus Creator/3
  q0-dot/1 -> Bus Creator/4
  Demux1/1 -> q0-dot/2
  Demux1/2 -> q1-dot/2
  Demux1/3 -> q2-dot/2
  Demux1/4 -> q3-dot/2
  Bus Creator/1 -> cek quaternion/1, Bus Selector/1, Bus Selector1/1
  Bus Selector/1 -> quaternion derivative/1(q0)  "<signal4>"
  Bus Selector/2 -> quaternion derivative/2(q1)  "<signal1>"
  Bus Selector/3 -> quaternion derivative/3(q2)  "<signal2>"
  Bus Selector/4 -> quaternion derivative/4(q3)  "<signal3>"
  Bus Selector1/1 -> Mux/1  "<signal4>"
  Bus Selector1/2 -> Mux/2  "<signal1>"
  Bus Selector1/3 -> Mux/3  "<signal2>"
  Bus Selector1/4 -> Mux/4  "<signal3>"

== system SatSIM_revAgustus16_01_R2013a/Environtments/Transformation Coordinate/ECEF to NED ==
  DCM RLG : Display
  Matrix Rotation ECEF to Local Horizon : MATLAB Function  TreatAsAtomicUnit=on
      settings: PermitHierarchicalResolution=ParametersOnly
  lat : Fcn  Expr=u(3)
  long : Fcn  Expr=u(3)
  rlg : Outport
  tag scope: RLG=global
  wires:
  Matrix Rotation ECEF to Local Horizon/1(Rlg) -> rlg/1, DCM RLG/1, [RLG]
  long/1 -> Matrix Rotation ECEF to Local Horizon/1(long)
  lat/1 -> Matrix Rotation ECEF to Local Horizon/2(lat)
  [Rt] -> lat/1, long/1

== system SatSIM_revAgustus16_01_R2013a/Environtments/Transformation Coordinate/ECEF to alt,lat,long ==
  Rt : Inport
  RGI : Inport  Port=2
  " " : MATLAB Function  TreatAsAtomicUnit=on
      settings: PermitHierarchicalResolution=ParametersOnly
  "   " : MATLAB Function  TreatAsAtomicUnit=on
      settings: PermitHierarchicalResolution=ParametersOnly
  Demux : Demux  Outputs=3
  Mux1 : Mux  Inputs=3
  T : Product  Multiplication=Matrix(*)
  alt,long,lat : MATLAB Function  TreatAsAtomicUnit=on
      settings: PermitHierarchicalResolution=ParametersOnly
  alt,lat,long : Outport
  wires:
  Mux1/1 -> alt,lat,long/1
  alt,long,lat/1(alt) -> Mux1/1
  "   "/1(longitude) -> Mux1/3
  " "/1(latitude) -> Mux1/2
  Demux/2 -> alt,long,lat/2(yG)
  alt,long,lat/3(lat) -> " "/1(lat)
  Demux/1 -> alt,long,lat/1(xG)
  T/1 -> Demux/1
  Demux/3 -> alt,long,lat/3(zG)
  alt,long,lat/2(long) -> "   "/1(long)
  RGI/1 -> T/1
  Rt/1 -> T/2

== system SatSIM_revAgustus16_01_R2013a/Environtments/Transformation Coordinate/ECI to ECEF ==
  DCM RGI : Display
  Matrix Rotation from ECI to ECEF : MATLAB Function  TreatAsAtomicUnit=on
      settings: PermitHierarchicalResolution=ParametersOnly
  teta : Display
  teta between ECT and ECEF : Subsystem
  rgi : Outport
  tag scope: RGI=global
  wires:
  teta between ECT and ECEF/1(teta) -> Matrix Rotation from ECI to ECEF/1(teta), teta/1
  [time] -> teta between ECT and ECEF/2(HMSt)
  [date] -> teta between ECT and ECEF/1(DMYt)
  Matrix Rotation from ECI to ECEF/1(Rgi) -> rgi/1, DCM RGI/1, [RGI]

== system SatSIM_revAgustus16_01_R2013a/Environtments/Transformation Coordinate/NED to ECI to Orbital ==
  Earth Magnetic Field (nT) in ECI : Display
  Earth Magnetic Field (nT) in Orbital Frame : Display
  T : Product  Multiplication=Matrix(*)
  T1 : Product  Multiplication=Matrix(*)
  b_obt : Scope
      settings: YMin=-27500  YMax=27500  SaveName=ScopeData7
  tag scope: b_eci=global, b_obt=global
  wires:
  [RIL] -> T/1
  T/1 -> [b_eci], T1/2, Earth Magnetic Field (nT) in ECI/1
  [b_ned] -> T/2
  T1/1 -> Earth Magnetic Field (nT) in Orbital Frame/1, [b_obt], b_obt/1
  [ROI] -> T1/1

== system SatSIM_revAgustus16_01_R2013a/Satellite Parameter INPUT/other parameter/Semi Major Axis and Semilatus Rectum ==
  E : Fcn  Expr=u(7)
  Mux : Mux  Inputs=2
  T (deg) : Display
  True Anomaly : Subsystem
  a and p : Display
  a n p : Subsystem
  e : Fcn  Expr=u(1)
  n : Fcn  Expr=u(5)
  tag scope: Tet=global, a=global, p=global
  wires:
  a n p/1(a) -> [a], Mux/1
  Mux/1 -> a and p/1
  [u] -> a n p/3(u)
  n/1 -> a n p/2(n)
  [obt_par] -> E/1, n/1, e/1
  a n p/2(p) -> [p], Mux/2
  e/1 -> True Anomaly/1(e), a n p/1(e)
  True Anomaly/1(T) -> [Tet], T (deg)/1
  E/1 -> True Anomaly/2(E)

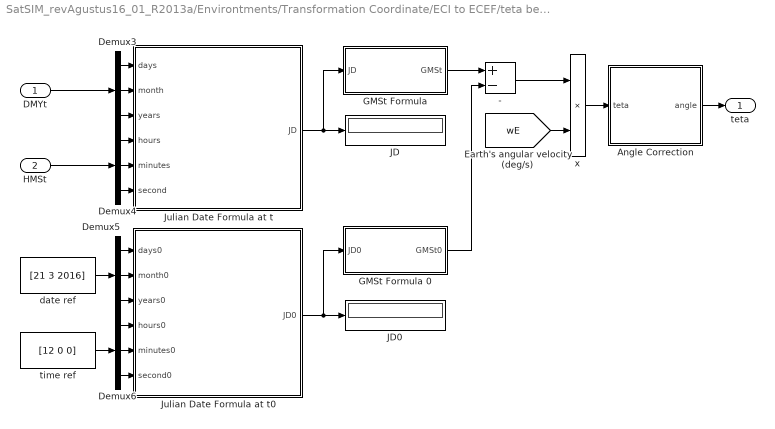
== system SatSIM_revAgustus16_01_R2013a/Environtments/Transformation Coordinate/ECI to ECEF/teta between ECT and ECEF ==
  DMYt : Inport
  HMSt : Inport  Port=2
  - : Sum  Inputs=+-
  Angle Correction : MATLAB Function  TreatAsAtomicUnit=on
      settings: PermitHierarchicalResolution=ParametersOnly
  Demux{3..6} (4 alike) : Demux  Outputs=3
  GMSt Formula : MATLAB Function  TreatAsAtomicUnit=on
      settings: PermitHierarchicalResolution=ParametersOnly
  GMSt Formula 0 : MATLAB Function  TreatAsAtomicUnit=on
      settings: PermitHierarchicalResolution=ParametersOnly
  JD : Display
  JD0 : Display
  Julian Date Formula at t : MATLAB Function  TreatAsAtomicUnit=on
      settings: PermitHierarchicalResolution=ParametersOnly
  Julian Date Formula at t0 : MATLAB Function  TreatAsAtomicUnit=on
      settings: PermitHierarchicalResolution=ParametersOnly
  date ref : Constant  Value=[21 3 2016]
  time ref : Constant  Value=[12 0 0]
  x : Product
  teta : Outport
  wires:
  GMSt Formula 0/1(GMSt0) -> -/2
  Julian Date Formula at t0/1(JD0) -> JD0/1, GMSt Formula 0/1(JD0)
  Julian Date Formula at t/1(JD) -> GMSt Formula/1(JD), JD/1
  Demux3/1 -> Julian Date Formula at t/1(days)
  Demux3/3 -> Julian Date Formula at t/3(years)
  DMYt/1 -> Demux3/1
  Demux6/2 -> Julian Date Formula at t0/5(minutes0)
  Demux5/2 -> Julian Date Formula at t0/2(month0)
  Demux6/3 -> Julian Date Formula at t0/6(second0)
  Demux6/1 -> Julian Date Formula at t0/4(hours0)
  Demux5/3 -> Julian Date Formula at t0/3(years0)
  Demux5/1 -> Julian Date Formula at t0/1(days0)
  -/1 -> x/1
  Demux4/1 -> Julian Date Formula at t/4(hours)
  HMSt/1 -> Demux4/1
  Demux4/2 -> Julian Date Formula at t/5(minutes)
  Demux4/3 -> Julian Date Formula at t/6(second)
  Demux3/2 -> Julian Date Formula at t/2(month)
  GMSt Formula/1(GMSt) -> -/1
  date ref/1 -> Demux5/1
  time ref/1 -> Demux6/1
  [wE] -> x/2
  x/1 -> Angle Correction/1(teta)
  Angle Correction/1(angle) -> teta/1

== system SatSIM_revAgustus16_01_R2013a/Satellite Parameter INPUT/other parameter/Semi Major Axis and Semilatus Rectum/True Anomaly ==
  note: 1-e
  note: 1+e
  e : Inport
  E : Inport  Port=2
  1 : Fcn  Expr=u(1)
  1+e/1-e : Product  Inputs=*/
  2 : Fcn  Expr=u(2)
  E/2 : Product  Inputs=*/
  Sqrt : Sqrt  SaturateOnIntegerOverflow=on
  Sum : Sum  Inputs=|++
  Sum1 : Sum  Inputs=|+-
  atan : Trigonometry  Operator=atan
  c : Constant  Value=[1 2]
  d2r : aerolibconvert2/Angle Conversion  IU=deg  OU=rad
  r2d : aerolibconvert2/Angle Conversion  IU=rad  OU=deg
  tan : Trigonometry  Operator=tan
  x : Product
  "x " : Product
  T : Outport
  wires:
  E/1 -> d2r/1
  atan/1 -> "x "/1
  1/1 -> Sum1/1, Sum/1
  c/1 -> 2/1, 1/1
  2/1 -> "x "/2, E/2/2
  E/2/1 -> tan/1
  Sum1/1 -> 1+e/1-e/2
  tan/1 -> x/2
  Sum/1 -> 1+e/1-e/1
  d2r/1 -> E/2/1
  1+e/1-e/1 -> Sqrt/1
  r2d/1 -> T/1
  e/1 -> Sum1/2, Sum/2
  x/1 -> atan/1
  Sqrt/1 -> x/1
  "x "/1 -> r2d/1

== system SatSIM_revAgustus16_01_R2013a/Satellite Parameter INPUT/other parameter/Semi Major Axis and Semilatus Rectum/a n p ==
  note: 1-e
  e : Inport
  n : Inport  Port=2
  u : Inport  Port=3
  1 : Fcn  Expr=u(1)
  1/c : Product  Inputs=*/
  1/d : Product  Inputs=*/
  2 : Fcn  Expr=u(2)
  Sum : Sum  Inputs=|+-
  c : Constant  Value=[1 2]
  pi : Constant  Value=1*pi
  sqr : Math  Operator=square  SaturateOnIntegerOverflow=on
  "sqr " : Math  Operator=square  SaturateOnIntegerOverflow=on
  sqrt3 : Fcn  Expr=u(1)^(1/3)
  t convert : Constant  Value=24*3600
  x : Product  Inputs=3
  "x " : Product
  a : Outport
  p : Outport  Port=2
  wires:
  "x "/1 -> p/1
  2/1 -> x/3
  1/c/1 -> "sqr "/1
  c/1 -> 1/1, 2/1
  n/1 -> x/1
  1/1 -> Sum/1
  sqrt3/1 -> "x "/2, a/1
  Sum/1 -> sqr/1
  u/1 -> 1/d/1
  sqr/1 -> "x "/1
  x/1 -> 1/c/1
  pi/1 -> x/2
  "sqr "/1 -> 1/d/2
  1/d/1 -> sqrt3/1
  t convert/1 -> 1/c/2
  e/1 -> Sum/2

== matlab function SatSIM_revAgustus16_01_R2013a/Environtments/Transformation Coordinate/ECI to ECEF/teta between ECT and ECEF/Angle Correction ==
  data: teta input; angle output
function angle = angle(teta)
%-------------------------------------------------------------------------%
% untuk sudut negatif dan positif
% jika sudut > 360 maka harus dikasi suatu coef. c
% jika sudut >-360 maka harus dikali suatu coef. c
%-------------------------------------------------------------------------%
if teta<0 %sudut negatif
    cn=teta/360; %coef
    if abs(cn)<1
        angle=teta;
    else
        angle=teta+(fix(cn)*360);
    end
else %sudut positif
    cp=teta/360; %coef
    if cp<1
        angle=teta;
    else
        angle=teta-(fix(cp)*360);
    end
end
%-------------------------------------------------------------------------%
end

== matlab function SatSIM_revAgustus16_01_R2013a/Actuator/currents X ==
  data: Imax input; Ia output; Ix input
function Ia = currents(Imax,Ix)
%#Currents filter
if Ix>(-1*Imax) && Ix<Imax
    Ia=Ix;
else
    if Ix>0 %positif
        Ia=Imax;
    else % negatif
        Ia=-1*Imax;
    end
end
end

== matlab function SatSIM_revAgustus16_01_R2013a/dynamic orbital/DCM to Euler Parameter ==
  data: DCM input; B output
function B   = DCM_to_EulerParatmeter( DCM )
%CONVERTION FROM DIREC COSINES MATRIX TO EULER PARAMETER
%   dcm has 3x3 dimention
%   euler parameter, a=euler axis, have 3x1 componen
%   and Teta=Euler angle, in degree
B=zeros(4,1);

%define R=Trace(DCM)
R=trace(DCM);

%define A=[r23-r32; r31-r13; r12-r21]
A=[DCM(2,3)-DCM(3,2);...
    DCM(3,1)-DCM(1,3);...
    DCM(1,2)-DCM(2,1)];

%euler angle, T
T=acosd((R-1)/2);

%euler axis, a
a=(1/2*sind(T))*A;

B(1)=T;
B(2)=a(1);
B(3)=a(2);
B(4)=a(3);

end

== matlab function SatSIM_revAgustus16_01_R2013a/Satellite Parameter INPUT/initial r and v/Orbital Parameter to Initial Position&Velocity ==
  data: p input; r output; e input; i input; O input; o input; nu input; truLon input; argLat input; lonPer input; mu input; v output
%----------------------- Begin Code Sequence -----------------------------%
% Purpose:                                                                %
% Convert a given set of Keplerian Orbital Elements to state vectors in   %
% in the ECI frame of reference                                           %
%                                                                         %
%-------------------------------------------------------------------------%
%                                                                         %
% Inputs:                                                                 %
%--------                                                                  
%p                      [1 x N]                         Semilatus Rectum
%                                                       (km)
%
%e                      [1 x N]                         Eccentricity Magnitude
%                                                       (unitless)
%
%i                      [1 x N]                         inclination
%                                                       (radians)
%
%O                      [1 x N]                         Right Ascention of
%                                                       the ascending node
%                                                       (radians)
%
%o                      [1 x N]                         Argument of perigee
%                                                       (radians)
%
%nu                     [1 x N]                         True Anomaly
%                                                       (radians)
%
%truLon                 [1 x N]                         True Longitude
%                                                       (radians)
%
%argLat                 [1 x N]                         Argument of Latitude
%                                                       (radians)
%
%lonPer                 [1 x N]                         Longitude of Periapse
%                                                       (radians)
%
%mu                     double                          Gravitational Constant
%                                                       Defaults to Earth if
%                                                       not specified
%
% Outputs:
%---------                                                                %
%r_ECI                  [3 x N]                         Position Vector in
%                                                       ECI coordinate
%                                                       frame of reference
%
%v_ECI                  [3 x N]                         Velocity vector in
%                                                       ECI coordinate
%                                                       frame of reference
%
% References:
%-------------
%Vallado,D. Fundamentals of Astrodynamics and Applications. 2007.
%
% Function Dependencies:
%------------------
%None
%------------------------------------------------------------------       %
% Programed by Darin Koblick  03-04-2012                                  %
%------------------------------------------------------------------       %
function [r,v] = orb2rv(p,e,i,O,o,nu,truLon,argLat,lonPer,mu)
%Make all inputs consistent w/ dimensions
p = p(:); e = e(:); i = i(:); O = O(:); o = o(:); nu = nu(:);
ietol = 1e-8;
idx = e < ietol & mod(i,pi) < ietol;
if any(idx); o(idx) = 0; O(idx) = 0; nu(idx) = truLon(idx); end
idx = e < ietol & mod(i,pi) > ietol;
if any(idx); o(idx) = 0; nu(idx) = argLat(idx); end
idx = e > ietol & mod(i,pi) < ietol;
if any(idx); O(idx) = 0; o(idx) = lonPer(idx); end
%Find rPQW and vPQW
rPQW = cat(2,p.*cos(nu)./(1 +e.*cos(nu)),p.*sin(nu)./(1+e.*cos(nu)),zeros(size(nu)));
vPQW = cat(2,-sqrt(mu./p).*sin(nu),sqrt(mu./p).*(e+cos(nu)),zeros(size(nu)));
%Create Transformation Matrix
PQW2IJK = NaN(3,3,size(p,1));
cO = cos(O); sO = sin(O); co = cos(o); so = sin(o); ci = cos(i); si = sin(i);
PQW2IJK(1,1,:) = cO.*co-sO.*so.*ci; PQW2IJK(1,2,:) = -cO.*so-sO.*co.*ci; PQW2IJK(1,3,:) = sO.*si;
PQW2IJK(2,1,:) = sO.*co+cO.*so.*ci; PQW2IJK(2,2,:) = -sO.*so+cO.*co.*ci; PQW2IJK(2,3,:) = -cO.*si;
PQW2IJK(3,1,:) = so.*si;            PQW2IJK(3,2,:) = co.*si;             PQW2IJK(3,3,:) = ci;
%Transform rPQW and vPQW to rECI and vECI
r = multiDimMatrixMultiply(PQW2IJK,rPQW)';  
v = multiDimMatrixMultiply(PQW2IJK,vPQW)';
end

function c = multiDimMatrixMultiply(a,b)
c = NaN(size(b));
c(:,1) = sum(bsxfun(@times,a(1,:,:),permute(b,[3 2 1])),2);
c(:,2) = sum(bsxfun(@times,a(2,:,:),permute(b,[3 2 1])),2);
c(:,3) = sum(bsxfun(@times,a(3,:,:),permute(b,[3 2 1])),2);
end

== matlab function SatSIM_revAgustus16_01_R2013a/Environtments/Transformation Coordinate/ECI to ECEF/Matrix Rotation from ECI to ECEF ==
  data: teta input; Rgi output
function Rgi = RGI(teta)
%#codegen
%Rgi=matric rotation from ECI to ECEF
R=[cosd(teta) sind(teta) 0;...
    -sind(teta) cosd(teta) 0;...
    0 0 1];
Rgi = R;

== matlab function SatSIM_revAgustus16_01_R2013a/dynamic inertial/DCM to Euler Parameter ==
  data: DCM input; B output
function B   = DCM_to_EulerParatmeter( DCM )
%CONVERTION FROM DIREC COSINES MATRIX TO EULER PARAMETER
%   dcm has 3x3 dimention
%   euler parameter, a=euler axis, have 3x1 componen
%   and Teta=Euler angle, in degree
B=zeros(4,1);

%define R=Trace(DCM)
R=trace(DCM);

%define A=[r23-r32; r31-r13; r12-r21]
A=[DCM(2,3)-DCM(3,2);...
    DCM(3,1)-DCM(1,3);...
    DCM(1,2)-DCM(2,1)];

%euler angle, T
T=acosd((R-1)/2);

%euler axis, a
a=(1/2*sind(T))*A;

B(1)=T;
B(2)=a(1);
B(3)=a(2);
B(4)=a(3);

end

== matlab function SatSIM_revAgustus16_01_R2013a/orbit par(t)/R(t) and V(t) to Orbital Parameter ==
  data: r input; a output; v input; mu input; eMag output; i output; O output; o output; nu output; truLon output; argLat output; lonPer output; p output
%----------------------- Begin Code Sequence -----------------------------%
% Purpose:                                                                %
% Convert a given set of state vectors in ECI reference frame to orbital  %
% elements.                                                               %
%-------------------------------------------------------------------------%
%                                                                         %
% Inputs:                                                                 %
%--------                                                                  
%r_ECI                  [3 x N]                         Position Vector in
%                                                       ECI coordinate
%                                                       frame of reference
%
%v_ECI                  [3 x N]                         Velocity vector in
%                                                       ECI coordinate
%                                                       frame of reference
%
%mu                     double                          Gravitational Constant
%                                                       Defaults to Earth if
%                                                       not specified
% Outputs:
%---------                                                                %
%a                      [1 x N]                         Semi-Major Axis
%                                                       (km)
%
%eMag                   [1 x N]                         Eccentricity
%                                                       (unitless)
%
%i                      [1 x N]                         inclination
%                                                       (radians)
%
%O                      [1 x N]                         Right Ascention of
%                                                       the ascending node
%                                                       (radians)
%
%o                      [1 x N]                         Argument of perigee
%                                                       (radians)
%
%M                      [1 x N]                         Mean Anomaly
%                                                       (radians)
%
%truLon                 [1 x N]                         True Longitude
%                                                       (radians)
%
%argLat                 [1 x N]                         Argument of Latitude
%                                                       (radians)
%
%lonPer                 [1 x N]                         Longitude of Periapse
%                                                       (radians)
%
%p                      [1 x N]                         Semilatus Rectum
%                                                       (km)
%
% References:
%-------------
%Vallado,D. Fundamentals of Astrodynamics and Applications. 2007.
%
% Function Dependencies:
%------------------
%None
%------------------------------------------------------------------       %
% Programed by Darin Koblick  03-04-2012                                  %
% Updated to address circular equatorial orbits       12/12/2013          %
%------------------------------------------------------------------       %
function [a,eMag,i,O,o,nu,truLon,argLat,lonPer,p] = rv2orb(r,v,mu)
%Specific angular momentum
h = cross(r,v);
n = cross(repmat([0;0;1],[1,size(r,2)]),h); nMag = sqrt(sum(n.^2,1));
vMag = sqrt(sum(v.^2,1)); 
rMag = sqrt(sum(r.^2,1)); 
hMag = sqrt(sum(h.^2,1));
e = (1./mu).*(bsxfun(@times,(vMag.^2 - mu./rMag),r) - bsxfun(@times,dot(r,v),v)); 
eMag = sqrt(sum(e.^2,1));
zeta = (vMag.^2)./2 - mu./rMag;

%semi major axis
a = -mu./(2.*zeta); 
p = a.*(1-eMag.^2); 

%Compute the angles
i = acos(h(3,:)./hMag); 
O = acos(n(1,:)./nMag);
o = acos(dot(n,e)./(nMag.*eMag));
nu = acos(dot(e,r)./(eMag.*rMag));
lonPer = acos(e(1,:)./eMag);
argLat = acos(dot(n,r)./(nMag.*rMag));
truLon = acos(r(1,:)./rMag);
%Account for those cases where satellite is in circular orbit
         O(n(1,:) == 0) = 0;
       o(dot(n,e) == 0) = 0;
    lonPer(e(1,:) == 0) = 0;
      nu(dot(e,r) == 0) = 0;
  argLat(dot(n,r) == 0) = 0;
%Apply Quadrant Checks to All Determined Angles
idx = n(2,:) < 0; if any(idx);  O(idx) = 2*pi - O(idx);  end
idx = e(3,:) < 0; if any(idx); o(idx) = 2*pi - o(idx); end
idx = dot(r,v) < 0; if any(idx); nu(idx) = 2*pi - nu(idx); end
idx = e(2,:) < 0; if any(idx); lonPer(idx) = 2*pi-lonPer(idx);  end
idx = r(3,:) < 0; if any(idx); argLat(idx) = 2*pi - argLat(idx); end
idx = r(2,:) < 0; if any(idx); truLon(idx) = 2*pi - truLon(idx); end
end

== matlab function SatSIM_revAgustus16_01_R2013a/dynamic orbital/Eulr Par to Quaternion ==
  data: teta input; a1 input; Q output; a2 input; a3 input
function Q   = EulrPar_to_Q( teta,a1,a2,a3 )
%CALCULATE QUATERNION FROM EULER PARAMETER
%   This program calculated quaternion if given an euler parameter\
%   Q = quaternion, have a component 
%   Q = [q0 q1 q2 q3]
%   and Euler parameter, a = Euler Axis, dimention 1x3
%                        teta = Euler Angle, degree

%Quaternion
Q=[cosd(teta/2); a1*sind(teta/2); a2*sind(teta/2); a3*sind(teta/2)];

end

== matlab function SatSIM_revAgustus16_01_R2013a/Environtments/Transformation Coordinate/ECI to ECEF/teta between ECT and ECEF/GMSt Formula ==
  data: JD input; GMSt output
function GMSt = GMSt(JD)
%#codegen
%GreenWich MeanSidereal Time or LST at GreenWich
%if give a UT (universal time)
%First, Calculate Julian Century or T
T=(JD-2451545)/36525;

%so, the GMSt given by
G=24110.54841+(T*8640184.812866)+((T^2)*0.093104)-((T^3)*0.0000062);
%in hours

GMSt = G;
